simulink model "DifferentialDriveMotionModelTemplate"  (R2021b)
settings: Solver=FixedStepAuto  StartTime=0.0  StopTime=inf  FixedStep=.1  RelTol=1e-3
libraries: robotlib x4
settings Model: Creator=gavin  LastModifiedBy=Gavin
settings OptimizationCC: EnhancedBackFolding=on  PassReuseOutputArgsAs=Individual arguments  ZeroExternalMemoryAtStartup=off  ZeroInternalMemoryAtStartup=off  MaxStackSize=64  OptimizeBlockOrder=speed  DifferentSizesBufferReuse=on  OptimizationCustomize=off  EfficientTunableParamExpr=on
settings DebuggingCC: ParameterTunabilityLossMsg=error
settings HardwareCC: ProdBitPerPointer=32  ProdBitPerSizeT=32  ProdBitPerPtrDiffT=32  ProdLargestAtomicFloat=None  ProdIntDivRoundTo=Undefined  ProdEndianess=Unspecified  ProdWordSize=32  ProdHWDeviceType=Generic->Unspecified (assume 32-bit Generic)  UseEmbeddedCoderFeatures=off
settings SFSimCC: MATLABDynamicMemAlloc=off
settings RTWCC: Description=Embedded Coder  SystemTargetFile=ert.tlc  HardwareBoard=Robot Operating System (ROS)  TLCOptions="-aInlineSetEventsForThisBaseRateFcn=TLC_FALSE -aSuppressMultiTaskScheduler=TLC_FALSE  -aRateBasedStepFcn=0"  TemplateMakefile=ert_default_tmf  Toolchain=Catkin  TargetLang=C++
settings CodeAppCC: ForceParamTrailComments=on  IgnoreCustomStorageClasses=off  OperatorAnnotations=on  SimulinkDataObjDesc=on  SFDataObjDesc=on  InsertBlockDesc=on
settings ERTTargetCC: SupportNonInlinedSFcns=on

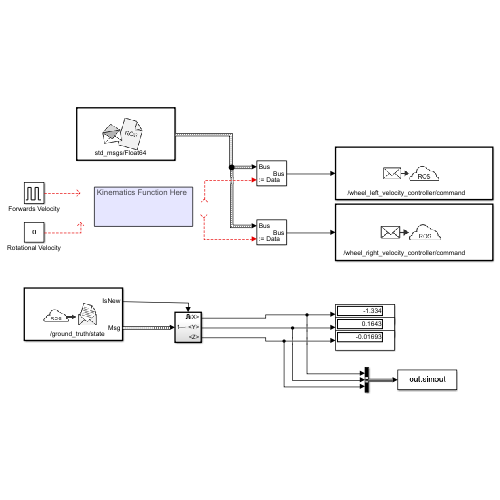
[thumbnail: Simulink's stored preview of the top-level diagram]
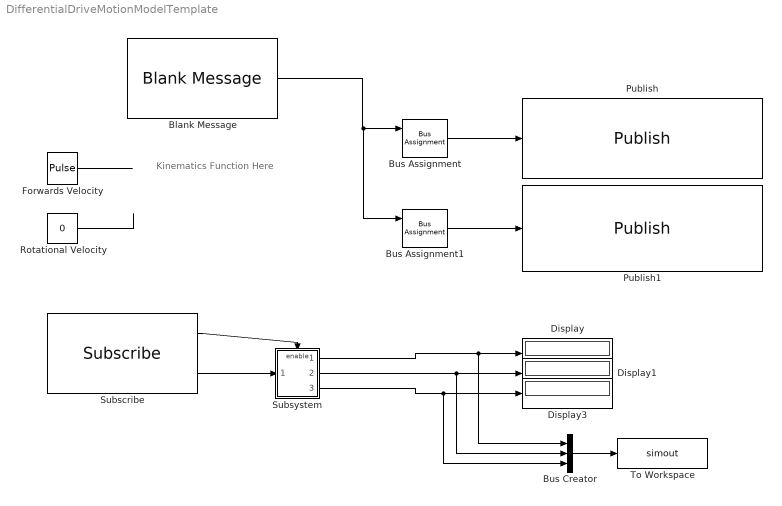
== system DifferentialDriveMotionModelTemplate ==
  note: Kinematics Function Here
  Blank Message : robotlib/Blank Message  messageClass=Message  entityType=std_msgs/Float64  messageType=std_msgs/Float64  SampleTime=-1  legacyBusStruct=off
  Bus Assignment : BusAssignment  AssignedSignals=Data
  Bus Assignment1 : BusAssignment  AssignedSignals=Data
  Bus Creator : BusCreator  Inputs=3
  Display : Display
  Display1 : Display
  Display3 : Display
  Forwards Velocity : DiscretePulseGenerator  PulseType=Time based  Amplitude=10  Period=10  PulseWidth=5
  Publish : robotlib/Publish  topicSource=Select from ROS network  topic=/wheel_left_velocity_controller/command  messageType=std_msgs/Float64  legacyBusStruct=off  messageQueueLength=1
  Publish1 : robotlib/Publish  topicSource=Select from ROS network  topic=/wheel_right_velocity_controller/command  messageType=std_msgs/Float64  legacyBusStruct=off  messageQueueLength=1
  Rotational Velocity : Constant  Value=0
  Subscribe : robotlib/Subscribe  topicSource=Select from ROS network  topic=/ground_truth/state  messageType=nav_msgs/Odometry  SampleTime=-1  legacyBusStruct=off  messageQueueLength=1
  Subsystem : Subsystem
  To Workspace : ToWorkspace  VariableName=simout  SaveFormat=Timeseries  SampleTime=-1
  wires:
  Blank Message/1 -> Bus Assignment1/1, Bus Assignment/1
  Subscribe/2 -> Subsystem/1(In1)
  Subsystem/1(<X>) -> Bus Creator/1, Display/1
  Subsystem/2(<Y>) -> Bus Creator/2, Display1/1
  Subsystem/3(<Z>) -> Bus Creator/3, Display3/1
  Subscribe/1 -> Subsystem/Enable
  Bus Creator/1 -> To Workspace/1
  Bus Assignment/1 -> Publish/1
  Bus Assignment1/1 -> Publish1/1
  ? -> Bus Assignment/2
  ? -> Bus Assignment1/2
  Forwards Velocity/1 -> ?
  Rotational Velocity/1 -> ?

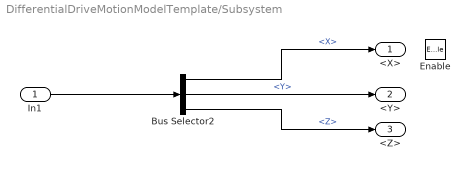
== system DifferentialDriveMotionModelTemplate/Subsystem ==
  In1 : Inport
  Enable : EnablePort
  Bus Selector2 : BusSelector  OutputSignals=Pose.Pose.Position.X,Pose.Pose.Position.Y,Twist.Twist.Angular.Z
  <X> : Outport
  <Y> : Outport  Port=2
  <Z> : Outport  Port=3
  wires:
  Bus Selector2/2 -> <Y>/1  "<Y>"
  In1/1 -> Bus Selector2/1
  Bus Selector2/1 -> <X>/1  "<X>"
  Bus Selector2/3 -> <Z>/1  "<Z>"
